simulink model "Team23_Pacemaker"  (R2020a)
settings: Solver=FixedStepAuto  StartTime=0.0  StopTime=10.0  FixedStep=1e-3  RelTol=1e-3  EnableMultiTasking=on
undefined symbols (not defined in the file): A0, A1, D0, D1, D10, D11, D12, D13, D2, D3, D4, D5, D6, D7, D8, D9, PTA0, PTA1, PTA2, PTB2, PTB23, PTB3, PTB9, PTC16, PTC17, PTC2, PTC3, PTC4, PTD0, PTD1, PTD2, PTD3
libraries: frdmk64flib x18
settings Model: ExtModeTrigDuration=5  Creator=Edward Xu  LastModifiedBy=Edward Xu
settings OptimizationCC: EnhancedBackFolding=on  PassReuseOutputArgsAs=Individual arguments  ZeroExternalMemoryAtStartup=off  ZeroInternalMemoryAtStartup=off  MaxStackSize=64  OptimizeBlockOrder=speed  DifferentSizesBufferReuse=on  OptimizationCustomize=off  EfficientTunableParamExpr=on
settings DebuggingCC: ParameterTunabilityLossMsg=error
settings HardwareCC: ProdBitPerPointer=32  ProdBitPerSizeT=32  ProdBitPerPtrDiffT=32  ProdLargestAtomicInteger=Long  ProdLargestAtomicFloat=Double  ProdWordSize=32  ProdHWDeviceType=ARM Compatible->ARM Cortex
settings SFSimCC: MATLABDynamicMemAlloc=off
settings RTWCC: SystemTargetFile=ert.tlc  HardwareBoard=NXP FRDM-K64F  TemplateMakefile=ert_default_tmf  Toolchain=GNU Tools for ARM Embedded Processors
settings CodeAppCC: ForceParamTrailComments=on  IgnoreCustomStorageClasses=off  OperatorAnnotations=on  SimulinkDataObjDesc=on  SFDataObjDesc=on  InsertBlockDesc=on

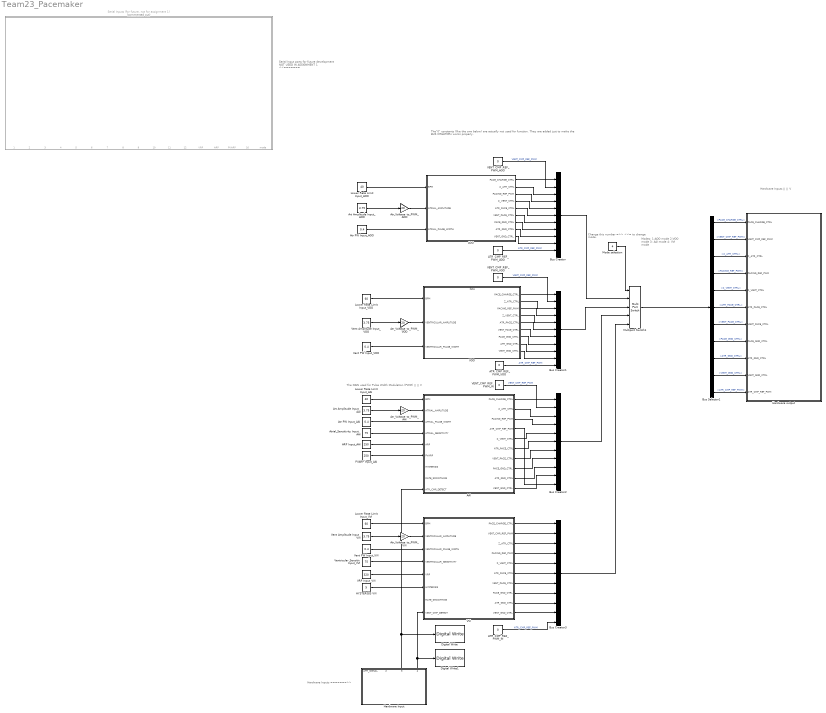
== system Team23_Pacemaker ==
  note: Change this number
      |
      | =>> <<=
      |
      | to change mode.
  note: Modes:
      | 1:AOO mode
      | 2:VOO mode
      | 3: AAI mode
      | 4: VVI mode
  note: Serial Input ports for future development
      | NOT USED IN ASSIGNMENT 1
      | <<=======
  note: Hardware Inputs
      | =======>>
  note: Hardware Inputs
      | ||
      | ||
      | V
  note: The"0" constants (like the one below) are actually not used for function.
      | They are added just to make the BUS CREATORs works properly.
  note: The GAIN used for Pulse Width Modulation (PWM)
      | ||
      | ||
      | V
  AAI : Stateflow chart  TreatAsAtomicUnit=on
      settings: PortSchema="{\"entries\":[{\"content\":{\"sides\":[{\"content\":{\"connectorIds\":[\"In1\",\"In2\",\"In3\",\"In4\",\"In5\",\"In6\",\"In7\",\"In8\",\"In9\"]},\"type\":\"ConnectorPlacement.EquallySpacedRectSide\",\"uuid\":\"b678de6f-9e61-4024-a0aa-5bf6d03f3d0b\"},{\"content\":{\"connectorIds\":[\"Out3\",\"Out8\",\"Out5\",\"Out10\",\"Out9\",\"Out2\",\"Out7\",\"Out4\",\"Out1\",\"Out6\"],\"side\":\"RIGHT\"},\"type\":\"ConnectorPlacement.EquallySpacedRectSide\",\"uuid\":\"4cd0faad-dd9d-4a56-81c5-44f7dd4bee31\"},{\"content\":{\"connectorIds\":[],\"side\":\"TOP\"},\"type\":\"ConnectorPlacement.EquallySpacedRectSide\",\"uuid\":\"a9bc4227-6f84-42c8-b827-a378e14304fe\"},{\"content\":{\"connectorIds\":[],\"side\":\"BOTTOM\"},\"type\":\"ConnectorPlacement.EquallySpacedRectSide\",\"uuid\":\"399184e4-c77f-47b0-89f0-adcbaf01dcf6\"}]},\"type\":\"ConnectorPlacement.EquallySpacedConnector\",\"uuid\":\"ee3b07ee-2423-4f21-89d4-53b7a563517d\"}],\"packageUris\":[\"http://schema.mathworks.com/mf0/Connector/19700101\"],\"version\":\"1.0\"}"
  AOO : Stateflow chart  TreatAsAtomicUnit=on
      settings: PortSchema="{\"entries\":[{\"content\":{\"sides\":[{\"content\":{\"connectorIds\":[\"In1\",\"In2\",\"In3\"]},\"type\":\"ConnectorPlacement.EquallySpacedRectSide\",\"uuid\":\"a22e05d8-b46e-41db-a99f-a3bab389e16c\"},{\"content\":{\"connectorIds\":[\"Out3\",\"Out8\",\"Out5\",\"Out9\",\"Out2\",\"Out7\",\"Out4\",\"Out1\",\"Out6\"],\"side\":\"RIGHT\"},\"type\":\"ConnectorPlacement.EquallySpacedRectSide\",\"uuid\":\"b830ec1d-656a-4b92-afcd-8fda6b31ad8a\"},{\"content\":{\"connectorIds\":[],\"side\":\"TOP\"},\"type\":\"ConnectorPlacement.EquallySpacedRectSide\",\"uuid\":\"956e5d71-b4a8-48ca-aae1-84adff4c1ec1\"}]},\"type\":\"ConnectorPlacement.EquallySpacedConnector\",\"uuid\":\"bd48be11-38ec-46b0-b71c-a53820608697\"}],\"packageUris\":[\"http://schema.mathworks.com/mf0/Connector/19700101\"],\"version\":\"1.0\"}"
  ARP Input_AAI : Constant  Value=250
  ATR_CMP_REF_PWM_AOO : Constant  Value=0
  ATR_CMP_REF_PWM_IN : Constant  Value=0
  ATR_CMP_REF_PWM_VOO : Constant  Value=0
  Art Amplitude Input_AAI : Constant  Value=3.75
  Art Amplitude Input_AOO : Constant  Value=3.75
  Atr PW Input_AAI : Constant  Value=0.4
  Atr PW Input_AOO : Constant  Value=0.4
  Atr_Voltage_to_PWM_AAI : Gain  Gain=20
  Atr_Voltage_to_PWM_AOO : Gain  Gain=20
  Atr_Voltage_to_PWM_VOO : Gain  Gain=20
  Atr_Voltage_to_PWM_VVI : Gain  Gain=20
  Atrial_Sensitivity Input_AAI : Constant  Value=75
  Bus Creator{,1..3} (4 alike) : BusCreator  Inputs=11
  Bus Selector1 : BusSelector  OutputSignals=PACE_CHARGE_CTRL,VENT_CMP_REF_PWM,Z_ATR_CTRL,PACING_REF_PWM,Z_VENT_CTRL,ATR_PACE_CTRL,VENT_PACE_CTRL,PACE_GND_CTRL,ATR_GND_CTRL,VENT_GND_CTRL,ATR_CMP_REF_PWM
  Digital Write : frdmk64flib/Digital Write  Whichpin=RED_LED
  Digital Write1 : frdmk64flib/Digital Write  Whichpin=BLUE_LED
  HYSTERISIS VVI : Constant  Value=5
  "Hardware Input " : Subsystem
      settings: PortSchema="{\"entries\":[{\"content\":{\"sides\":[{\"content\":{\"connectorIds\":[]},\"type\":\"ConnectorPlacement.EquallySpacedRectSide\",\"uuid\":\"a4541679-de89-4a95-8b75-854a44d8a186\"},{\"content\":{\"connectorIds\":[],\"side\":\"RIGHT\"},\"type\":\"ConnectorPlacement.EquallySpacedRectSide\",\"uuid\":\"6fd79412-9f15-416b-b660-00aa28626d8b\"},{\"content\":{\"connectorIds\":[\"Out1\",\"Out2\",\"Out3\",\"Out4\"],\"side\":\"TOP\"},\"type\":\"ConnectorPlacement.EquallySpacedRectSide\",\"uuid\":\"ae8cadce-7179-46b5-afab-b52bf988a3ac\"}]},\"type\":\"ConnectorPlacement.EquallySpacedConnector\",\"uuid\":\"277cb13a-90c8-489f-9404-664107ee015d\"}],\"packageUris\":[\"http://schema.mathworks.com/mf0/Connector/19700101\"],\"version\":\"1.0\"}"
  Hardware output : Subsystem
  Lower Rate Limit Input_AAI : Constant  Value=40
  Lower Rate Limit Input_AOO : Constant  Value=40
  Lower Rate Limit Input_VOO : Constant  Value=60
  Lower Rate Limit Input_VVI : Constant  Value=60
  Mode selection : Constant  Value=4
  Multiport Switch1 : MultiPortSwitch  Inputs=4  DiagnosticForDefault=Warning
  PVARP Input_AAI : Constant  Value=250
  "Serial Inputs (for future, not for assignment 1)" : Subsystem  Commented=on
      settings: PortSchema="{\"entries\":[{\"content\":{\"sides\":[{\"content\":{\"connectorIds\":[]},\"type\":\"ConnectorPlacement.EquallySpacedRectSide\",\"uuid\":\"703cf520-d471-4fb9-b1b3-e5ef227936b0\"},{\"content\":{\"connectorIds\":[],\"side\":\"RIGHT\"},\"type\":\"ConnectorPlacement.EquallySpacedRectSide\",\"uuid\":\"164fb1c9-5e01-45a9-8906-aed3049631a5\"},{\"content\":{\"connectorIds\":[],\"side\":\"TOP\"},\"type\":\"ConnectorPlacement.EquallySpacedRectSide\",\"uuid\":\"65caf497-dd89-4d28-be0b-91bb62c499fd\"},{\"content\":{\"connectorIds\":[\"Out1\",\"Out2\",\"Out3\",\"Out4\",\"Out5\",\"Out6\",\"Out7\",\"Out8\",\"Out9\",\"Out10\",\"Out11\",\"Out12\",\"Out13\",\"Out14\",\"Out15\",\"Out16\",\"Out17\"],\"side\":\"BOTTOM\"},\"type\":\"ConnectorPlacement.EquallySpacedRectSide\",\"uuid\":\"2d54c024-7d22-4a04-894c-ab2b45ca92fe\"}]},\"type\":\"ConnectorPlacement.EquallySpacedConnector\",\"uuid\":\"c9a4482e-8c58-4eb3-90e0-1d102ae6fa0f\"}],\"packageUris\":[\"http://schema.mathworks.com/mf0/Connector/19700101\"],\"version\":\"1.0\"}"
  VENT_CMP_REF_PWM_AOO : Constant  Value=0
  VENT_CMP_REF_PWM_IN : Constant  Value=0
  VENT_CMP_REF_PWM_VOO : Constant  Value=0
  VOO : Stateflow chart  TreatAsAtomicUnit=on
      settings: PortSchema="{\"entries\":[{\"content\":{\"sides\":[{\"content\":{\"connectorIds\":[\"In2\",\"In3\",\"In4\"]},\"type\":\"ConnectorPlacement.EquallySpacedRectSide\",\"uuid\":\"a22e05d8-b46e-41db-a99f-a3bab389e16c\"},{\"content\":{\"connectorIds\":[\"Out3\",\"Out8\",\"Out5\",\"Out9\",\"Out2\",\"Out7\",\"Out4\",\"Out1\",\"Out6\"],\"side\":\"RIGHT\"},\"type\":\"ConnectorPlacement.EquallySpacedRectSide\",\"uuid\":\"b830ec1d-656a-4b92-afcd-8fda6b31ad8a\"},{\"content\":{\"connectorIds\":[\"In1\"],\"side\":\"TOP\"},\"type\":\"ConnectorPlacement.EquallySpacedRectSide\",\"uuid\":\"956e5d71-b4a8-48ca-aae1-84adff4c1ec1\"}]},\"type\":\"ConnectorPlacement.EquallySpacedConnector\",\"uuid\":\"bd48be11-38ec-46b0-b71c-a53820608697\"}],\"packageUris\":[\"http://schema.mathworks.com/mf0/Connector/19700101\"],\"version\":\"1.0\"}"
  VRP Input_VVI : Constant  Value=320
  VVI : Stateflow chart  TreatAsAtomicUnit=on
      settings: PortSchema="{\"entries\":[{\"content\":{\"sides\":[{\"content\":{\"connectorIds\":[\"In1\",\"In2\",\"In3\",\"In4\",\"In5\",\"In6\",\"In7\",\"In8\"]},\"type\":\"ConnectorPlacement.EquallySpacedRectSide\",\"uuid\":\"b678de6f-9e61-4024-a0aa-5bf6d03f3d0b\"},{\"content\":{\"connectorIds\":[\"Out3\",\"Out10\",\"Out8\",\"Out5\",\"Out9\",\"Out2\",\"Out7\",\"Out4\",\"Out1\",\"Out6\"],\"side\":\"RIGHT\"},\"type\":\"ConnectorPlacement.EquallySpacedRectSide\",\"uuid\":\"4cd0faad-dd9d-4a56-81c5-44f7dd4bee31\"},{\"content\":{\"connectorIds\":[],\"side\":\"TOP\"},\"type\":\"ConnectorPlacement.EquallySpacedRectSide\",\"uuid\":\"a9bc4227-6f84-42c8-b827-a378e14304fe\"},{\"content\":{\"connectorIds\":[],\"side\":\"BOTTOM\"},\"type\":\"ConnectorPlacement.EquallySpacedRectSide\",\"uuid\":\"d9bc86ca-c62d-429e-b855-d0c137c2bc24\"}]},\"type\":\"ConnectorPlacement.EquallySpacedConnector\",\"uuid\":\"ee3b07ee-2423-4f21-89d4-53b7a563517d\"}],\"packageUris\":[\"http://schema.mathworks.com/mf0/Connector/19700101\"],\"version\":\"1.0\"}"
  Vent Amplitude Input_VOO : Constant  Value=3.75
  Vent Amplitude Input_VVI : Constant  Value=3.75
  Vent PW Input_VOO : Constant  Value=0.4
  Vent PW Input_VVI : Constant  Value=0.4
  Ventricular_Sensitiy Input_VVI : Constant  Value=75
  wires:
  AOO/3(PACE_CHARGE_CTRL) -> Bus Creator/1
  AOO/8(Z_ATR_CTRL) -> Bus Creator/3
  AOO/5(PACING_REF_PWM) -> Bus Creator/4
  AOO/9(Z_VENT_CTRL) -> Bus Creator/5
  AOO/2(ATR_PACE_CTRL) -> Bus Creator/6
  AOO/7(VENT_PACE_CTRL) -> Bus Creator/7
  AOO/4(PACE_GND_CTRL) -> Bus Creator/8
  AOO/1(ATR_GND_CTRL) -> Bus Creator/9
  AOO/6(VENT_GND_CTRL) -> Bus Creator/10
  VENT_CMP_REF_PWM_IN/1 -> Bus Creator2/2  "VENT_CMP_REF_PWM"
  ATR_CMP_REF_PWM_IN/1 -> Bus Creator3/11  "ATR_CMP_REF_PWM"
  VVI/7(VENT_PACE_CTRL) -> Bus Creator3/7
  AAI/7(VENT_PACE_CTRL) -> Bus Creator2/7
  VVI/9(Z_VENT_CTRL) -> Bus Creator3/5
  AAI/4(PACE_GND_CTRL) -> Bus Creator2/8
  AAI/1(ATR_GND_CTRL) -> Bus Creator2/9
  VVI/8(Z_ATR_CTRL) -> Bus Creator3/3
  VOO/3(PACE_CHARGE_CTRL) -> Bus Creator1/1
  AAI/3(PACE_CHARGE_CTRL) -> Bus Creator2/1
  VOO/6(VENT_GND_CTRL) -> Bus Creator1/10
  VOO/1(ATR_GND_CTRL) -> Bus Creator1/9
  VVI/10(VENT_CMP_REF_PWM) -> Bus Creator3/2
  AAI/8(Z_ATR_CTRL) -> Bus Creator2/3
  AAI/2(ATR_PACE_CTRL) -> Bus Creator2/6
  VOO/9(Z_VENT_CTRL) -> Bus Creator1/5
  VVI/4(PACE_GND_CTRL) -> Bus Creator3/8
  VVI/3(PACE_CHARGE_CTRL) -> Bus Creator3/1
  VVI/2(ATR_PACE_CTRL) -> Bus Creator3/6
  VOO/8(Z_ATR_CTRL) -> Bus Creator1/3
  VOO/2(ATR_PACE_CTRL) -> Bus Creator1/6
  VVI/5(PACING_REF_PWM) -> Bus Creator3/4
  VVI/1(ATR_GND_CTRL) -> Bus Creator3/9
  VOO/5(PACING_REF_PWM) -> Bus Creator1/4
  VOO/7(VENT_PACE_CTRL) -> Bus Creator1/7
  AAI/10(ATR_CMP_REF_PWM) -> Bus Creator2/11
  VVI/6(VENT_GND_CTRL) -> Bus Creator3/10
  AAI/6(VENT_GND_CTRL) -> Bus Creator2/10
  VOO/4(PACE_GND_CTRL) -> Bus Creator1/8
  AAI/5(PACING_REF_PWM) -> Bus Creator2/4
  AAI/9(Z_VENT_CTRL) -> Bus Creator2/5
  "Hardware Input "/3(ATR_CMP_DETECT) -> Digital Write/1, AAI/9(ATR_CMP_DETECT)
  "Hardware Input "/4(VENT_CMP_DETECT) -> Digital Write1/1, VVI/8(VENT_CMP_DETECT)
  Bus Selector1/1 -> Hardware output/1(PACE_CHARGE_CTRL)  "<PACE_CHARGE_CTRL>"
  Bus Selector1/2 -> Hardware output/2(VENT_CMP_REF_PWM)  "<VENT_CMP_REF_PWM>"
  Bus Selector1/3 -> Hardware output/3(Z_ATR_CTRL)  "<Z_ATR_CTRL>"
  Bus Selector1/4 -> Hardware output/4(PACING_REF_PWM)  "<PACING_REF_PWM>"
  Multiport Switch1/1 -> Bus Selector1/1
  Bus Creator2/1 -> Multiport Switch1/4
  Bus Creator1/1 -> Multiport Switch1/3
  Bus Creator3/1 -> Multiport Switch1/5
  ATR_CMP_REF_PWM_AOO/1 -> Bus Creator/11  "ATR_CMP_REF_PWM"
  VENT_CMP_REF_PWM_AOO/1 -> Bus Creator/2  "VENT_CMP_REF_PWM"
  Bus Creator/1 -> Multiport Switch1/2
  Bus Selector1/5 -> Hardware output/5(Z_VENT_CTRL)  "<Z_VENT_CTRL>"
  Bus Selector1/6 -> Hardware output/6(ATR_PACE_CTRL)  "<ATR_PACE_CTRL>"
  Bus Selector1/7 -> Hardware output/7(VENT_PACE_CTRL)  "<VENT_PACE_CTRL>"
  Bus Selector1/8 -> Hardware output/8(PACE_GND_CTRL)  "<PACE_GND_CTRL>"
  Bus Selector1/9 -> Hardware output/9(ATR_GND_CTRL)  "<ATR_GND_CTRL>"
  Bus Selector1/10 -> Hardware output/10(VENT_GND_CTRL)  "<VENT_GND_CTRL>"
  Bus Selector1/11 -> Hardware output/11(ATR_CMP_REF_PWM)  "<ATR_CMP_REF_PWM>"
  Lower Rate Limit Input_AAI/1 -> AAI/1(BPM)
  Art Amplitude Input_AAI/1 -> Atr_Voltage_to_PWM_AAI/1
  Atr_Voltage_to_PWM_AAI/1 -> AAI/2(ATRIAL_AMPLITUDE)
  Atr PW Input_AAI/1 -> AAI/3(ATRIAL_PULSE_WIDTH)
  Atrial_Sensitivity Input_AAI/1 -> AAI/4(ATRIAL_SENSITIVITY)
  ARP Input_AAI/1 -> AAI/5(ARP)
  PVARP Input_AAI/1 -> AAI/6(PVARP)
  Vent PW Input_VOO/1 -> VOO/4(VENTRICULAR_PULSE_WIDTH)
  Lower Rate Limit Input_VOO/1 -> VOO/2(BPM)
  Vent Amplitude Input_VOO/1 -> Atr_Voltage_to_PWM_VOO/1
  Atr PW Input_AOO/1 -> AOO/3(ATRIAL_PULSE_WIDTH)
  Lower Rate Limit Input_AOO/1 -> AOO/1(BPM)
  Art Amplitude Input_AOO/1 -> Atr_Voltage_to_PWM_AOO/1
  Atr_Voltage_to_PWM_VOO/1 -> VOO/3(VENTRICULAR_AMPLITUDE)
  Atr_Voltage_to_PWM_AOO/1 -> AOO/2(ATRIAL_AMPLITUDE)
  Lower Rate Limit Input_VVI/1 -> VVI/1(BPM)
  Vent PW Input_VVI/1 -> VVI/3(VENTRICULAR_PULSE_WIDTH)
  Ventricular_Sensitiy Input_VVI/1 -> VVI/4(VENTRICULAR_SENSITIVITY)
  Vent Amplitude Input_VVI/1 -> Atr_Voltage_to_PWM_VVI/1
  Atr_Voltage_to_PWM_VVI/1 -> VVI/2(VENTRICULAR_AMPLITUDE)
  VRP Input_VVI/1 -> VVI/5(VRP)
  Mode selection/1 -> Multiport Switch1/1
  VENT_CMP_REF_PWM_VOO/1 -> Bus Creator1/2  "VENT_CMP_REF_PWM"
  ATR_CMP_REF_PWM_VOO/1 -> Bus Creator1/11  "ATR_CMP_REF_PWM"
  HYSTERISIS VVI/1 -> VVI/6(HYSTERISIS)

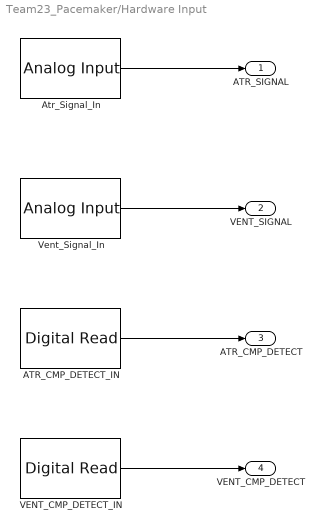
== system Team23_Pacemaker/Hardware Input  ==
  ATR_CMP_DETECT_IN : frdmk64flib/Digital Read  Whichpin=PTC16 (D0)  SampleTime=-1
  Atr_Signal_In : frdmk64flib/Analog Input  Whichpin=PTB2 (A0)  SampleTime=-1
  VENT_CMP_DETECT_IN : frdmk64flib/Digital Read  Whichpin=PTC17 (D1)  SampleTime=-1
  Vent_Signal_In : frdmk64flib/Analog Input  Whichpin=PTB3 (A1)  SampleTime=-1
  ATR_SIGNAL : Outport
  VENT_SIGNAL : Outport  Port=2
  ATR_CMP_DETECT : Outport  Port=3  OutDataTypeStr=boolean
  VENT_CMP_DETECT : Outport  Port=4  OutDataTypeStr=boolean
  wires:
  VENT_CMP_DETECT_IN/1 -> VENT_CMP_DETECT/1
  ATR_CMP_DETECT_IN/1 -> ATR_CMP_DETECT/1
  Vent_Signal_In/1 -> VENT_SIGNAL/1
  Atr_Signal_In/1 -> ATR_SIGNAL/1

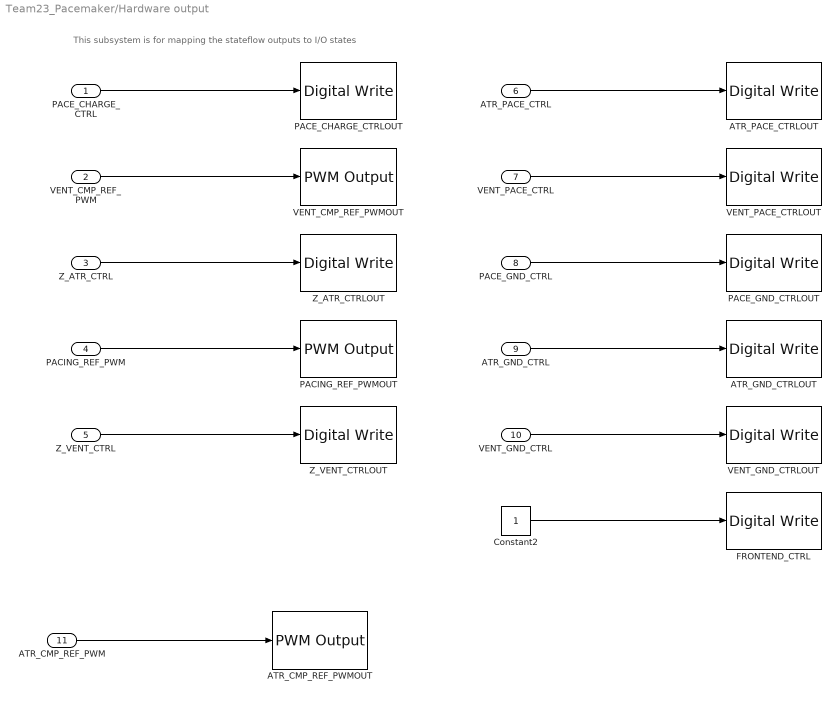
== system Team23_Pacemaker/Hardware output ==
  note: This subsystem is for mapping the stateflow outputs to I/O states
  PACE_CHARGE_CTRL : Inport
  VENT_CMP_REF_PWM : Inport  Port=2
  Z_ATR_CTRL : Inport  Port=3
  PACING_REF_PWM : Inport  Port=4
  Z_VENT_CTRL : Inport  Port=5
  ATR_PACE_CTRL : Inport  Port=6
  VENT_PACE_CTRL : Inport  Port=7
  PACE_GND_CTRL : Inport  Port=8
  ATR_GND_CTRL : Inport  Port=9
  VENT_GND_CTRL : Inport  Port=10
  ATR_CMP_REF_PWM : Inport  Port=11
  ATR_CMP_REF_PWMOUT : frdmk64flib/PWM Output  Whichpin=PTC2 (D6)  InitialFrequency=2000  InitialDutyCycle=0
  ATR_GND_CTRLOUT : frdmk64flib/Digital Write  Whichpin=PTD2 (D11)
  ATR_PACE_CTRLOUT : frdmk64flib/Digital Write  Whichpin=PTA0 (D8)
  Constant2 : Constant
  FRONTEND_CTRL : frdmk64flib/Digital Write  Whichpin=PTD1 (D13)
  PACE_CHARGE_CTRLOUT : frdmk64flib/Digital Write  Whichpin=PTB9 (D2)
  PACE_GND_CTRLOUT : frdmk64flib/Digital Write  Whichpin=PTD0 (D10)
  PACING_REF_PWMOUT : frdmk64flib/PWM Output  Whichpin=PTA2 (D5)  InitialFrequency=2000  InitialDutyCycle=0
  VENT_CMP_REF_PWMOUT : frdmk64flib/PWM Output  Whichpin=PTA1 (D3)  InitialFrequency=2000  InitialDutyCycle=0
  VENT_GND_CTRLOUT : frdmk64flib/Digital Write  Whichpin=PTD3 (D12)
  VENT_PACE_CTRLOUT : frdmk64flib/Digital Write  Whichpin=PTC4 (D9)
  Z_ATR_CTRLOUT : frdmk64flib/Digital Write  Whichpin=PTB23 (D4)
  Z_VENT_CTRLOUT : frdmk64flib/Digital Write  Whichpin=PTC3 (D7)
  wires:
  Z_VENT_CTRL/1 -> Z_VENT_CTRLOUT/1
  Z_ATR_CTRL/1 -> Z_ATR_CTRLOUT/1
  ATR_CMP_REF_PWM/1 -> ATR_CMP_REF_PWMOUT/1
  VENT_GND_CTRL/1 -> VENT_GND_CTRLOUT/1
  PACE_CHARGE_CTRL/1 -> PACE_CHARGE_CTRLOUT/1
  VENT_PACE_CTRL/1 -> VENT_PACE_CTRLOUT/1
  Constant2/1 -> FRONTEND_CTRL/1
  PACE_GND_CTRL/1 -> PACE_GND_CTRLOUT/1
  ATR_GND_CTRL/1 -> ATR_GND_CTRLOUT/1
  PACING_REF_PWM/1 -> PACING_REF_PWMOUT/1
  ATR_PACE_CTRL/1 -> ATR_PACE_CTRLOUT/1
  VENT_CMP_REF_PWM/1 -> VENT_CMP_REF_PWMOUT/1

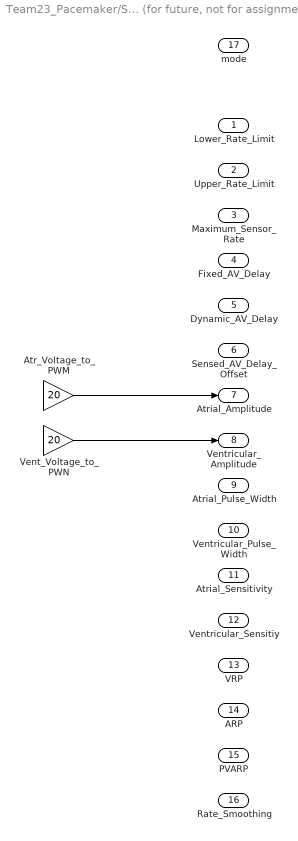
== system Team23_Pacemaker/Serial Inputs (for future, not for assignment 1) ==
  Atr_Voltage_to_PWM : Gain  Gain=20
  Vent_Voltage_to_PWN : Gain  Gain=20
  Lower_Rate_Limit : Outport
  Upper_Rate_Limit : Outport  Port=2
  Maximum_Sensor_Rate : Outport  Port=3
  Fixed_AV_Delay : Outport  Port=4
  Dynamic_AV_Delay : Outport  Port=5
  Sensed_AV_Delay_Offset : Outport  Port=6
  Atrial_Amplitude : Outport  Port=7
  Ventricular_Amplitude : Outport  Port=8
  Atrial_Pulse_Width : Outport  Port=9
  Ventricular_Pulse_Width : Outport  Port=10
  Atrial_Sensitivity : Outport  Port=11
  Ventricular_Sensitiy : Outport  Port=12
  VRP : Outport  Port=13
  ARP : Outport  Port=14
  PVARP : Outport  Port=15
  Rate_Smoothing : Outport  Port=16
  mode : Outport  Port=17
  wires:
  Vent_Voltage_to_PWN/1 -> Ventricular_Amplitude/1
  Atr_Voltage_to_PWM/1 -> Atrial_Amplitude/1

== stateflow chart Team23_Pacemaker/VVI ==
  note: VVI will only pace the ventricle if the natural heartbeat drops below that of the defined lower limit
  state INIT
    entry:
    VENT_CMP_REF_PWM = VENTRICULAR_SENSITIVITY;
    PACING_REF_PWM = VENTRICULAR_AMPLITUDE;
    ATR_GND_CTRL = 0;
    ATR_PACE_CTRL = 0;
    Z_ATR_CTRL = 0;
    Z_VENT_CTRL = 0;
    PACE_GND_CTRL = 1;
    last_pulse_natural = false;
  state DISCHARGE
    entry:
    VENT_PACE_CTRL = 0;
    VENT_GND_CTRL = 1;
  state PULSE_VENT
    entry:
    PACE_CHARGE_CTRL = 0;
    VENT_GND_CTRL = 0;
    VENT_PACE_CTRL = 1;
  state CHARGE
    entry:
    VENT_PACE_CTRL = 0;
    PACE_CHARGE_CTRL = 1;
  state PULSE_SET_NATURAL
    entry:
    last_pulse_natural = true;
  state PULSE_SET_ARTIFICIAL
    entry:
    last_pulse_natural = false;
  note: skip pulse if natural heart beat is detected
  note: Something wrong with this poor guy's heart
      | START PACING THE VENTRICLE!!!
  state hold
    entry:
  (default) -> INIT
  DISCHARGE -> INIT
  PULSE_VENT -> DISCHARGE : after(VENTRICULAR_PULSE_WIDTH, msec)
  INIT -> CHARGE
  PULSE_SET_ARTIFICIAL -> PULSE_VENT
  PULSE_SET_NATURAL -> CHARGE
  hold -> PULSE_SET_NATURAL [order 1] : [VENT_CMP_DETECT == 1]
  CHARGE -> hold : after(VRP, msec)
  hold -> PULSE_SET_ARTIFICIAL [order 2] : after(60000/BPM-VENTRICULAR_PULSE_WIDTH-VRP, msec)[ last_pulse_natural == false || HYSTERISIS == 0]
  data: ATR_GND_CTRL output; ATR_PACE_CTRL output; PACE_CHARGE_CTRL output; PACE_GND_CTRL output; PACING_REF_PWM output; VENT_GND_CTRL output; VENT_PACE_CTRL output; Z_ATR_CTRL output; Z_VENT_CTRL output; BPM input; VENTRICULAR_AMPLITUDE input; VENTRICULAR_PULSE_WIDTH input; VENTRICULAR_SENSITIVITY input; VRP input; HYSTERISIS input; RATE_SMOOTHING input; VENT_CMP_REF_PWM output; VENT_CMP_DETECT input; last_pulse_natural local

== stateflow chart Team23_Pacemaker/AAI ==
  note: AAI will only pace the atrium if the natural heartbeat drops below that of the defined lower limit
  state INIT
    entry:
    ATR_CMP_REF_PWM = ATRIAL_SENSITIVITY;
    PACING_REF_PWM = ATRIAL_AMPLITUDE;
    VENT_GND_CTRL = 0;
    VENT_PACE_CTRL = 0;
    Z_ATR_CTRL = 0;
    Z_VENT_CTRL = 0;
    PACE_GND_CTRL = 1;
    last_pulse_natural = false;
  state DISCHARGE
    entry:
    ATR_PACE_CTRL = 0;
    ATR_GND_CTRL = 1;
  state CHARGE
    entry:
    ATR_PACE_CTRL = 0;
    PACE_CHARGE_CTRL = 1;
  state PULSE_SET_NATURAL
    entry:
    last_pulse_natural = true;
  note: skip pulse if natural heart beat is detected
  state PULSE_ATR
    entry:
    PACE_CHARGE_CTRL = 0;
    ATR_GND_CTRL = 0;
    ATR_PACE_CTRL = 1;
  state hold
    entry:
  note: Something wrong with this poor guy's heart
      | START PACING THE ATRIUM!!!
  state PULSE_SET_ARTIFICIAL
    entry:
    last_pulse_natural = false;
  DISCHARGE -> INIT
  (default) -> INIT
  PULSE_ATR -> DISCHARGE : after(ATRIAL_PULSE_WIDTH, msec)
  INIT -> CHARGE
  PULSE_SET_NATURAL -> CHARGE
  hold -> PULSE_SET_NATURAL [order 1] : [ATR_CMP_DETECT == 1]
  CHARGE -> hold : after(ARP, msec)
  hold -> PULSE_SET_ARTIFICIAL [order 3] : after(60000/(BPM-HYSTERISIS)-ARP, msec)[ last_pulse_natural == true && HYSTERISIS > 0]
  hold -> PULSE_SET_ARTIFICIAL [order 2] : after(60000/BPM-ARP, msec)[ last_pulse_natural == false || HYSTERISIS == 0]
  PULSE_SET_ARTIFICIAL -> PULSE_ATR
  data: ATR_GND_CTRL output; ATR_PACE_CTRL output; PACE_CHARGE_CTRL output; PACE_GND_CTRL output; PACING_REF_PWM output; VENT_GND_CTRL output; VENT_PACE_CTRL output; Z_ATR_CTRL output; Z_VENT_CTRL output; BPM input; ATRIAL_AMPLITUDE input; ATRIAL_PULSE_WIDTH input; ATRIAL_SENSITIVITY input; ARP input; PVARP input; HYSTERISIS input; RATE_SMOOTHING input; last_pulse_natural local; ATR_CMP_DETECT input; ATR_CMP_REF_PWM output

== stateflow chart Team23_Pacemaker/VOO ==
  note: VOO mode paces the ventricle at a constant rate regardless of the natural heartbeat
  state CHARGE
    entry:
    ATR_PACE_CTRL = 0;
    VENT_PACE_CTRL = 0;
    PACING_REF_PWM = VENTRICULAR_AMPLITUDE;
    PACE_CHARGE_CTRL = 1;
  state PULSE_VENT
    entry:
    PACE_CHARGE_CTRL = 0;
    PACE_GND_CTRL = 1;
    ATR_PACE_CTRL = 0;
    ATR_GND_CTRL = 0;
    Z_ATR_CTRL = 0;
    Z_VENT_CTRL = 0;
    VENT_GND_CTRL = 0;
    VENT_PACE_CTRL = 1;
  state DISCHARGE
    entry:
    PACE_GND_CTRL = 1;
    VENT_PACE_CTRL = 0;
    Z_ATR_CTRL = 0;
    Z_VENT_CTRL = 0;
    ATR_PACE_CTRL = 0;
    ATR_GND_CTRL = 0;
    VENT_GND_CTRL = 1;
  (default) -> CHARGE
  CHARGE -> PULSE_VENT : after(60/BPM,sec)
  DISCHARGE -> CHARGE
  PULSE_VENT -> DISCHARGE : after(VENTRICULAR_PULSE_WIDTH, msec)
  data: data input; ATR_GND_CTRL output; ATR_PACE_CTRL output; PACE_CHARGE_CTRL output; PACE_GND_CTRL output; PACING_REF_PWM output; VENT_GND_CTRL output; VENT_PACE_CTRL output; Z_ATR_CTRL output; Z_VENT_CTRL output; BPM input; VENTRICULAR_AMPLITUDE input; VENTRICULAR_PULSE_WIDTH input

== stateflow chart Team23_Pacemaker/AOO ==
  note: AOO mode paces the atrium at a constant rate regardless of the natural heartbeat
  state CHARGE
    entry:
    ATR_PACE_CTRL = 0;
    VENT_PACE_CTRL = 0;
    PACING_REF_PWM = ATRIAL_AMPLITUDE;
    PACE_CHARGE_CTRL = 1;
  state PULSE_ATR
    entry:
    PACE_CHARGE_CTRL = 0;
    PACE_GND_CTRL = 1;
    VENT_GND_CTRL = 0;
    VENT_PACE_CTRL = 0;
    Z_ATR_CTRL = 0;
    Z_VENT_CTRL = 0;
    ATR_GND_CTRL = 0;
    ATR_PACE_CTRL = 1;
  state DISCHARGE
    entry:
    PACE_GND_CTRL = 1;
    VENT_PACE_CTRL = 0;
    Z_ATR_CTRL = 0;
    Z_VENT_CTRL = 0;
    ATR_PACE_CTRL = 0;
    ATR_GND_CTRL = 0;
    VENT_GND_CTRL = 1;
  (default) -> CHARGE
  CHARGE -> PULSE_ATR : after(60/BPM,sec)
  DISCHARGE -> CHARGE
  PULSE_ATR -> DISCHARGE : after(ATRIAL_PULSE_WIDTH, msec)
  data: ATR_GND_CTRL output; ATR_PACE_CTRL output; PACE_CHARGE_CTRL output; PACE_GND_CTRL output; PACING_REF_PWM output; VENT_GND_CTRL output; VENT_PACE_CTRL output; Z_ATR_CTRL output; Z_VENT_CTRL output; BPM input; ATRIAL_AMPLITUDE input; ATRIAL_PULSE_WIDTH input
